simulink model "TP2_retour_simple"  (R2024a)
settings: Solver=VariableStepAuto  StartTime=0.0  StopTime=10.0  RelTol=1e-3
undefined symbols (not defined in the file): A, B1, B2, C, C1
libraries: spspowerguiLib x1
settings Model: Creator=hp  LastModifiedBy=NB
settings SolverCC: AlgebraicLoopSolver=TrustRegion
settings DataIOCC: ReturnWorkspaceOutputs=off
settings DebuggingCC: UnconnectedInputMsg=warning  UnconnectedOutputMsg=warning  UnconnectedLineMsg=warning  ArithmeticOperatorsInVariantConditions=warning
settings ModelReferenceCC: EnableRefExpFcnMdlSchedulingChecks=on
settings SFSimCC: CustomCodeUndefinedFunction=UseInterfaceOnly
settings RTWCC: GPUComputeCapability=3.5

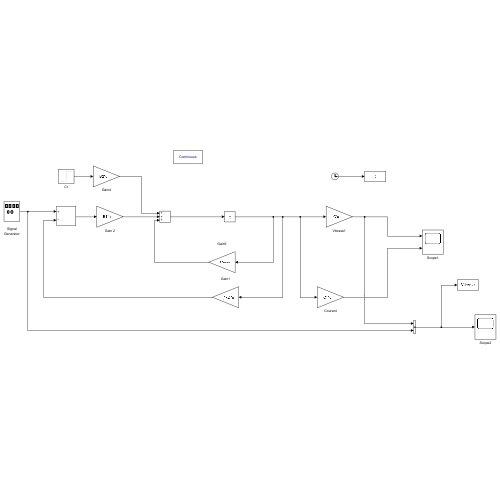
[thumbnail: Simulink's stored preview of the top-level diagram]
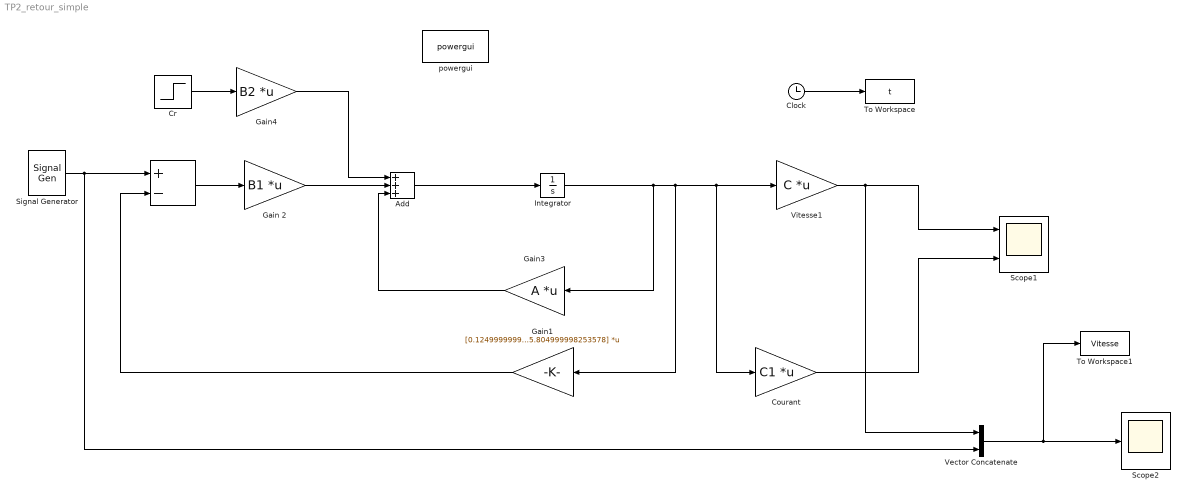
== system TP2_retour_simple ==
  " " : Sum  Inputs=+-
  " Signal Generator" : SignalGenerator  WaveForm=square  Amplitude=12  Frequency=0.25
  Add : Sum  Inputs=+++
  Clock : Clock
  "Courant " : Gain  Gain=C1  Multiplication=Matrix(K*u)
  Cr : Step  After=0  SampleTime=0
  "Gain 2 " : Gain  Gain=B1  Multiplication=Matrix(K*u)
  "Gain1 " : Gain  Gain=[0.124999999978977,25.804999998253578]  Multiplication=Matrix(K*u)
  "Gain3 " : Gain  Gain=A  Multiplication=Matrix(K*u) (u vector)
  "Gain4 " : Gain  Gain=B2  Multiplication=Matrix(K*u)
  Integrator : Integrator
  "Scope1 " : Scope  NumInputPorts=2
  "Scope2 " : Scope
  To Workspace : ToWorkspace  VariableName=t  SaveFormat=Timeseries  SampleTime=-1
  To Workspace1 : ToWorkspace  VariableName=Vitesse  SaveFormat=Timeseries  SampleTime=-1
  Vector Concatenate : Concatenate
  "Vitesse1 " : Gain  Gain=C  Multiplication=Matrix(K*u)
  powergui : spspowerguiLib/powergui  Priority=1  SimulationMode=Continuous  SampleTime=50e-6  frequency=60  Iterations=50  frequencyindice=60  Pbase=100e6  ErrMax=1e-4  UnitsV=kV  UnitsW=MW  buscounter=0  FunctionMessages=off  echomessages=off  EnableUseOfTLC=off  CurrentSourceSwitches=off  DisableSnubberDevices=off  DisableRonSwitches=off  DisableVfSwitches=off  DisplayEquations=off  AutomaticDiscreteSolvers=off  SolverType=Tustin/Backward Euler (TBE)  Interpol=off  ExternalGateDelay=off  methode=off  Ts=100  x0status=blocks  SPID=on  SwTol=0  HookPort=off  NonlinearTolerance=1e-4  nMaxIteration=100  ContinueOnMaxIteration=off  RestoreLinks=warning  ResistiveCurrentMeasurement=off  Frange=[0:2:500]  Ylog=off  Xlog=on  ShowGrid=off  save=off  variable=ZData  structure=0  ZoomFFT=off  StartTime=0.0  cycles=1  DisplayStyle=1  fundamental=60  FreqAxis=off  MaxFrequency=1000  frequencyindicesteady=1  RmsSteady=1  display=off
  wires:
  Integrator/1 -> "Gain3 "/1, "Gain1 "/1, "Courant "/1, "Vitesse1 "/1
  "Vitesse1 "/1 -> Vector Concatenate/1, "Scope1 "/1
  "Courant "/1 -> "Scope1 "/2
  Vector Concatenate/1 -> To Workspace1/1, "Scope2 "/1
  " "/1 -> "Gain 2 "/1
  "Gain1 "/1 -> " "/2
  Cr/1 -> "Gain4 "/1
  " Signal Generator"/1 -> Vector Concatenate/2, " "/1
  Clock/1 -> To Workspace/1
  "Gain3 "/1 -> Add/3
  "Gain 2 "/1 -> Add/2
  "Gain4 "/1 -> Add/1
  Add/1 -> Integrator/1
